simulink model "Lead_Acid_Battery2"  (R2024b)
settings: Solver=VariableStepAuto  StartTime=0.0  StopTime=36000  RelTol=1e-3
settings Model: Creator=10537  LastModifiedBy=10537

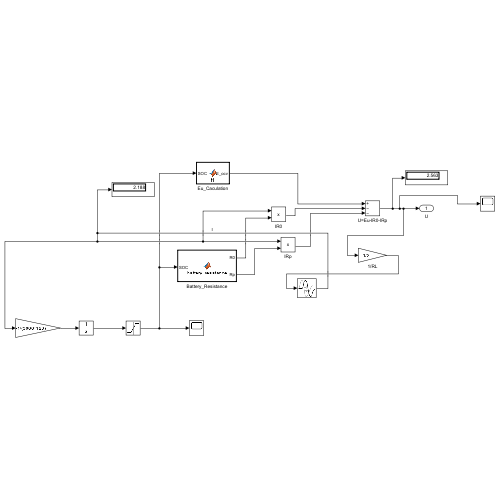
[thumbnail: Simulink's stored preview of the top-level diagram]
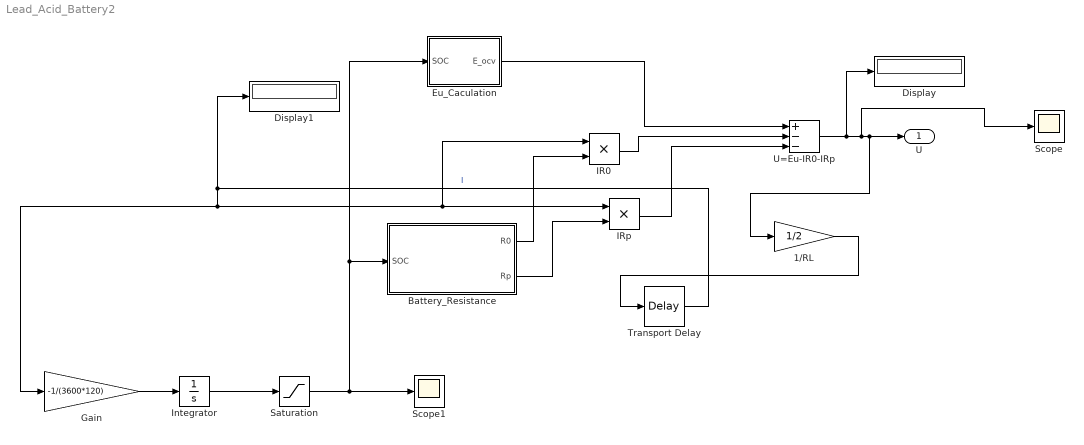
== system Lead_Acid_Battery2 ==
  1/RL : Gain  Gain=1/2
  Battery_Resistance : MATLAB Function  TreatAsAtomicUnit=on
  Display : Display
  Display1 : Display
  Eu_Caculation : MATLAB Function  TreatAsAtomicUnit=on
  Gain : Gain  Gain=-1/(3600*120)
  IR0 : Product
  IRp : Product
  Integrator : Integrator  InitialCondition=0.9
  Saturation : Saturate  UpperLimit=1  LowerLimit=0
  Scope : Scope
  Scope1 : Scope
  Transport Delay : TransportDelay  DelayTime=1e-5  InitialOutput=200
  U=Eu-IR0-IRp : Sum  Inputs=+--
  U : Outport
  wires:
  Eu_Caculation/1(E_ocv) -> U=Eu-IR0-IRp/1
  Transport Delay/1 -> Gain/1, IRp/1, IR0/1, Display1/1  "I"
  IR0/1 -> U=Eu-IR0-IRp/2
  Battery_Resistance/2(Rp) -> IRp/2
  Battery_Resistance/1(R0) -> IR0/2
  IRp/1 -> U=Eu-IR0-IRp/3
  U=Eu-IR0-IRp/1 -> Display/1, Scope/1, 1/RL/1, U/1
  1/RL/1 -> Transport Delay/1
  Gain/1 -> Integrator/1
  Integrator/1 -> Saturation/1
  Saturation/1 -> Scope1/1, Eu_Caculation/1(SOC), Battery_Resistance/1(SOC)

== matlab function Lead_Acid_Battery2/Battery_Resistance ==
  data: SOC input; R0 output; Rp output
function [R0, Rp] = battery_resistance(SOC)
    % 电池的欧姆内阻 R0（根据二次曲线拟合）
    a0 = 0.5; a1 = 0.1; a2 = -0.02;  
    R0 = a0 + a1 * SOC + a2 * SOC^2;

    % 电池的极化内阻 Rp（根据指数曲线拟合）
    b0 = 0.05; b1 = 3; b2 = 0.01;  
    Rp = b0 * exp(-b1 * SOC) + b2;
end

== matlab function Lead_Acid_Battery2/Eu_Caculation ==
  data: SOC input; E_ocv output
function E_ocv = f1(SOC)
    % 电池的开路电压E_ocv与SOC的多项式关系
    E_ocv = 3.7 * SOC^3 - 0.8 * SOC^2 + 2.1 * SOC + 1.0;  % 拟合多项式
end
